simulink model "CubeSatTEST"  (R2024b)
settings: Solver=ode4  StartTime=simul.t0  StopTime=simul.tf  FixedStep=0.01  RelTol=1e-3
values from neighbouring files (symbols this model uses):
  alpha1 = 0.7    [mainSimTEST.m]
  alpha2 = 0.3    [mainSimTEST.m]
undefined symbols (not defined in the file or in its folder): act, DiscIntNeverNeededParam, env, flag, IC, K, orb, sat, sens
libraries: matrix_library x55, simulink_extras x5, simulink x2
(part 5 of 10)

== system CubeSatTEST/Real World/DKE (Dynamics Kinematics Environment)/Environment/Perturbations/Magnetic Field Torque ==
  r_n : Inport
  A(B/N) : Inport  Port=2
  Clock : Clock
  Constant : Constant  Value=env.mag.dgrf2020
  Constant1 : Constant  Value=env.Earth.R
  Constant2 : Constant  Value=3
  Constant3 : Constant  Value=env.Earth.magInclination
  Constant4 : Constant  Value=3
  Constant5 : Constant  Value=flag.mag
  Constant6 : Constant  Value=[0; 0; 0]
  Constant7 : Constant  Value=sat.jB
  Cos : Trigonometry  Operator=cos
  Cos1 : Trigonometry  Operator=cos
  Cross Product : matrix_library/Cross Product
  Divide : Product  Inputs=***/
  Divide1 : Product  Inputs=*/
  Divide2 : Product  Inputs=*/
  Dot Product : DotProduct  OutDataTypeStr=Inherit: Inherit via internal rule
  Gain : Gain  Gain=3
  Gain1 : Gain  Gain=env.Earth.omega
  Mux : Mux  Inputs=3
  Norm : Subsystem
  Norm1 : Subsystem
  Norm2 : Subsystem
  Power : Math  Operator=pow
  Power1 : Math  Operator=pow
  Product : Product
  Product1 : Product
  Product2 : Product
  Product9 : Product  Multiplication=Matrix(*)
  Sin : Trigonometry
  Sin1 : Trigonometry
  Sqrt : Sqrt
  Square : Math  Operator=square
  Subtract : Sum  Inputs=+-
  Sum of Elements : Sum  Inputs=+
  Switch : Switch  Criteria=u2 > Threshold  SaturateOnIntegerOverflow=off  InputSameDT=off
  T_mag : Outport
  wires:
  Constant/1 -> Square/1
  Square/1 -> Sum of Elements/1
  Sum of Elements/1 -> Sqrt/1
  Constant1/1 -> Power/1
  Constant2/1 -> Power/2
  Sqrt/1 -> Divide/2
  Power/1 -> Divide/3
  Constant4/1 -> Power1/2
  Power1/1 -> Divide/4
  Norm/1(Norm) -> Power1/1  "norm_r"
  r_n/1 -> Norm2/1(Vector), Divide2/1, [rr]
  [rr] -> Norm/1(Vector)
  [rr_hat] -> Dot Product/2
  Subtract/1 -> Divide/1
  [mm] -> Subtract/2
  Dot Product/1 -> Product/2
  Product/1 -> Gain/1
  Gain/1 -> Subtract/1
  [rr_hat] -> Product/1
  [mm] -> Dot Product/1
  Mux/1 -> Norm1/1(Vector), Divide1/1
  Cos/1 -> Mux/3
  Constant3/1 -> Sin/1, Cos/1
  Clock/1 -> Gain1/1
  Sin/1 -> Product2/2, Product1/2
  Product1/1 -> Mux/2
  Product2/1 -> Mux/1
  Cos1/1 -> Product2/1
  Gain1/1 -> Cos1/1, Sin1/1
  Sin1/1 -> Product1/1
  Divide/1 -> Product9/2
  Norm1/1(Norm) -> Divide1/2  "norm_r"
  Divide1/1 -> [mm]
  Norm2/1(Norm) -> Divide2/2  "norm_r"
  Divide2/1 -> [rr_hat]
  Constant5/1 -> Switch/2
  Constant6/1 -> Switch/3
  Cross Product/1 -> Switch/1
  A(B/N)/1 -> Product9/1
  Constant7/1 -> Cross Product/1
  Switch/1 -> T_mag/1
  Product9/1 -> Cross Product/2

== system CubeSatTEST/Real World/DKE (Dynamics Kinematics Environment)/Environment/Perturbations/Solar Radiation Pressure Torque ==
  S_b : Inport
  Constant : Constant  Value=flag.srp
  Constant1 : Constant  Value=[0; 0; 0]
  Constant3 : Constant  Value=ones(6,1)-sat.rho_s
  Constant4 : Constant  Value=sat.rho_s
  Constant5 : Constant  Value=sat.rho_d
  Gain1 : Gain  Gain=-env.dis.P
  Gain2 : Gain  Gain=2
  Gain3 : Gain  Gain=2/3
  Matrix Concatenate : Concatenate  NumInputs=3  Mode=Multidimensional array
  Matrix Concatenate2 : Concatenate  NumInputs=3  Mode=Multidimensional array
  MatrixMultiply : Product  Multiplication=Matrix(*)
  Normaliser : Subsystem
  Product{,1,3..4} (4 alike) : Product
  Product2 : Product  Multiplication=Matrix(*)
  Reshape : Reshape
  Saturation : Saturate  UpperLimit=1  LowerLimit=0
  Sum1 : Sum  Inputs=+|+
  Sum2 : Sum  Inputs=+|+
  Switch : Switch  Criteria=u2 > Threshold  SaturateOnIntegerOverflow=off  InputSameDT=off
  Transpose : Math  Operator=transpose
  Transpose2 : Math  Operator=transpose
  Transpose3 : Math  Operator=transpose
  cross product r x F : Subsystem
  surface : Constant  Value=sat.A
  unit vector matrix : Constant  Value=sat.n_b
  T_srp : Outport
  wires:
  Product3/1 -> Transpose3/1
  Saturation/1 -> Product4/2, Product1/1
  Gain3/1 -> Sum1/2
  surface/1 -> Gain1/1
  unit vector matrix/1 -> MatrixMultiply/2, Product/2
  Constant4/1 -> Gain2/1
  Constant3/1 -> Product2/1
  Sum2/1 -> Product3/2
  [S_b] -> Product2/2
  Constant5/1 -> Gain3/1
  Product4/1 -> Sum1/1
  MatrixMultiply/1 -> Saturation/1
  Gain2/1 -> Product4/1
  Product2/1 -> Transpose/1
  S_b/1 -> Normaliser/1(Vector)
  Normaliser/1(Out1) -> Transpose2/1
  Transpose2/1 -> MatrixMultiply/1, [S_b]
  Product/1 -> Sum2/2
  Transpose/1 -> Sum2/1
  Transpose3/1 -> cross product r x F/1(F_srp)
  Gain1/1 -> Product1/2
  Sum1/1 -> Matrix Concatenate/3, Matrix Concatenate/1, Matrix Concatenate/2
  Matrix Concatenate/1 -> Product/1
  Product1/1 -> Matrix Concatenate2/3, Matrix Concatenate2/2, Matrix Concatenate2/1
  Matrix Concatenate2/1 -> Product3/1
  cross product r x F/1(Out1) -> Switch/1
  Constant/1 -> Switch/2
  Switch/1 -> Reshape/1
  Constant1/1 -> Switch/3
  Reshape/1 -> T_srp/1

== system CubeSatTEST/Real World/DKE (Dynamics Kinematics Environment)/Environment/Sun Direction Circular Orbit/Normaliser (with Built In safety) ==
  Vector : Inport
  Constant : Constant  Value=[0; 0; 0]  VectorParams1D=off
  Norm1 : Subsystem
  Protected Division : Subsystem
  Switch : Switch  Criteria=u2 ~= 0  SaturateOnIntegerOverflow=off  InputSameDT=off
  Out1 : Outport
  wires:
  Norm1/1(Norm) -> Switch/2, Protected Division/2(Norm)  "norm_r"
  Switch/1 -> Out1/1
  Protected Division/1(Out1) -> Switch/1
  Vector/1 -> Protected Division/1(Vector), Norm1/1(Vector)
  Constant/1 -> Switch/3

== system CubeSatTEST/Real World/DKE (Dynamics Kinematics Environment)/Kinematics/EulerKinematicsdelay/312 Propagator ==
  IC : Inport
  w_b : Inport  Port=2
  Reset : Inport  Port=3
  Cos1 : Trigonometry  Operator=cos
  Cos2 : Trigonometry  Operator=cos
  Demux : Demux  Outputs=3
  Demux1 : Demux  Outputs=3
  Divide1 : Product  Inputs=*/
  Integrator1 : Integrator  ExternalReset=either  InitialConditionSource=external  WrapState=on  WrappedStateUpperValue=2*pi  WrappedStateLowerValue=0  ShowStatePort=on
  Integrator2 : Integrator  ExternalReset=either  InitialConditionSource=external  WrapState=on  ShowStatePort=on
  Integrator3 : Integrator  ExternalReset=either  InitialConditionSource=external  WrapState=on  WrappedStateUpperValue=2*pi  WrappedStateLowerValue=0  ShowStatePort=on
  Mux : Mux  Inputs=3
  Mux1 : Mux  Inputs=3
  Product{1..7} (7 alike) : Product
  Sin : Trigonometry
  Subtract : Sum  Inputs=+-
  Subtract1 : Sum
  Subtract2 : Sum  Inputs=+-
  Subtract3 : Sum  Inputs=+-
  Tan : Trigonometry  Operator=tan
  EA : Outport
  Out1 : Outport  Port=2
  wires:
  Product6/1 -> Subtract3/2
  Product5/1 -> Subtract3/1
  Product4/1 -> Subtract1/2
  Integrator3/1 -> [theta3]
  [wz] -> Product5/1
  Mux/1 -> EA/1
  Product7/1 -> Subtract2/2
  Cos1/1 -> [cosPsi]
  [theta3] -> Sin/1, Cos1/1
  [cosPsi] -> Product1/2
  Demux/2 -> [wy]
  Tan/1 -> [tanThe]
  Product2/1 -> Subtract/2
  [wz] -> Product3/1
  [tanThe] -> Product7/2
  Cos2/1 -> [cosThe]
  [cosPsi] -> Product5/2
  Divide1/1 -> Integrator1/1
  Subtract1/1 -> Integrator2/1
  Demux/3 -> [wz]
  [theta1] -> Mux/1
  Subtract/1 -> Divide1/1
  Demux/1 -> [wx]
  Subtract2/1 -> Integrator3/1
  [theta2] -> Tan/1, Cos2/1
  [wy] -> Subtract2/1
  Integrator1/1 -> [theta1]
  Integrator2/1 -> [theta2]
  [wx] -> Product4/1
  [sinPsi] -> Product2/2
  w_b/1 -> Demux/1
  Subtract3/1 -> Product7/1
  Product3/1 -> Subtract1/1
  [theta2] -> Mux/2
  [sinPsi] -> Product3/2
  [theta3] -> Mux/3
  [sinPsi] -> Product6/2
  [wx] -> Product6/1
  [wx] -> Product2/1
  [cosPsi] -> Product4/2
  [wz] -> Product1/1
  Product1/1 -> Subtract/1
  [cosThe] -> Divide1/2
  Sin/1 -> [sinPsi]
  Demux1/1 -> Integrator1/3
  Demux1/2 -> Integrator2/3
  Demux1/3 -> Integrator3/3
  IC/1 -> Demux1/1
  Reset/1 -> Integrator2/2, Integrator3/2, Integrator1/2
  Integrator3/State -> Mux1/3
  Integrator2/State -> Mux1/2
  Integrator1/State -> Mux1/1
  Mux1/1 -> Out1/1

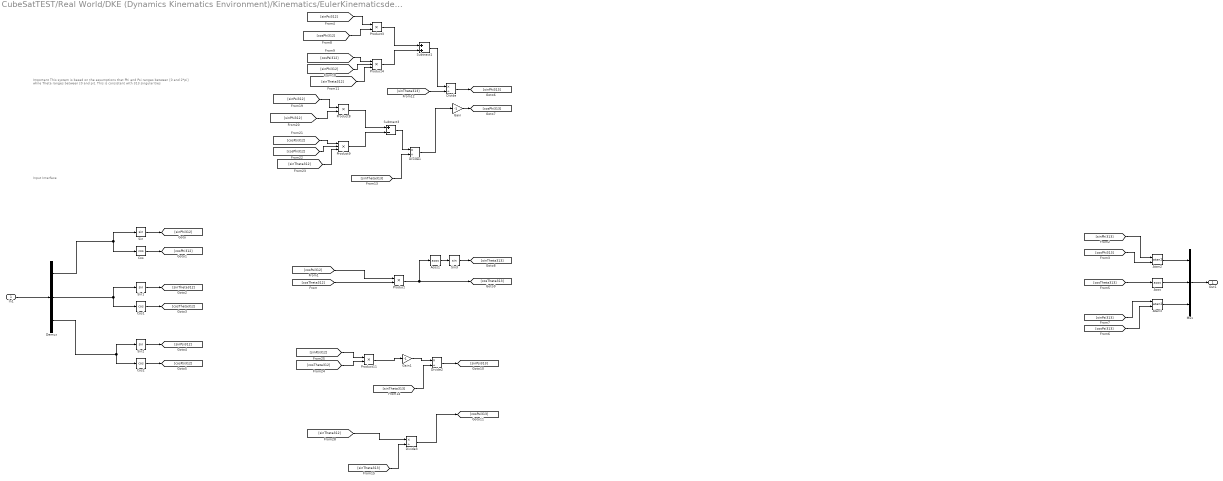
== system CubeSatTEST/Real World/DKE (Dynamics Kinematics Environment)/Kinematics/EulerKinematicsdelay/312To313 ==
  note: Important
      |
      | This system is based on the assumptions that Phi and Psi ranges between [0 and 2*pi] while Theta ranges between [0 and pi]. This is consistent with 313 singularities
  note: Input Interface
  In1 : Inport
  Acos : Trigonometry  Operator=acos
  Acos1 : Trigonometry  Operator=acos
  Atan2 : Trigonometry  Operator=atan2
  Atan3 : Trigonometry  Operator=atan2
  Cos : Trigonometry  Operator=cos
  Cos1 : Trigonometry  Operator=cos
  Cos2 : Trigonometry  Operator=cos
  Demux : Demux  Outputs=3
  Divide{,1..3} (4 alike) : Product  Inputs=*/
  Gain : Gain  Gain=-1
  Gain1 : Gain  Gain=-1
  Mux : Mux  Inputs=3
  Product{,3,8,11} (4 alike) : Product
  Product4 : Product  Inputs=3
  Product9 : Product  Inputs=3
  Sin{,1..3} (4 alike) : Trigonometry
  Subtract1 : Sum
  Subtract3 : Sum  Inputs=+-
  Out1 : Outport
  wires:
  In1/1 -> Demux/1
  Mux/1 -> Out1/1
  Sin/1 -> [sinPhi312]
  Cos/1 -> [cosPhi312]
  Demux/1 -> Sin/1, Cos/1
  Sin1/1 -> [sinTheta312]
  Demux/2 -> Sin1/1, Cos1/1
  Cos1/1 -> [cosTheta312]
  Sin2/1 -> [sinPsi312]
  Cos2/1 -> [cosPsi312]
  Demux/3 -> Sin2/1, Cos2/1
  Product/1 -> Acos1/1, [cosTheta313]
  [cosTheta312] -> Product/2
  [cosPsi312] -> Product/1
  Atan2/1 -> Mux/1
  Acos/1 -> Mux/2
  Atan3/1 -> Mux/3
  [sinPhi313] -> Atan2/1
  [cosPhi313] -> Atan2/2
  [cosTheta313] -> Acos/1
  [cosPsi313] -> Atan3/2
  [sinPsi313] -> Atan3/1
  Sin3/1 -> [sinTheta313]
  Acos1/1 -> Sin3/1
  [cosPsi312] -> Product4/1
  [sinTheta312] -> Product4/3
  Product3/1 -> Subtract1/1
  [cosPhi312] -> Product3/2
  Product4/1 -> Subtract1/2
  [sinPsi312] -> Product3/1
  [sinPhi312] -> Product4/2
  Divide/1 -> [sinPhi313]
  [sinTheta313] -> Divide/2
  Subtract1/1 -> Divide/1
  Gain/1 -> [cosPhi313]
  Divide1/1 -> Gain/1
  [sinTheta313] -> Divide1/2
  [cosPsi312] -> Product9/1
  Product9/1 -> Subtract3/2
  Subtract3/1 -> Divide1/1
  [sinPsi312] -> Product8/1
  [cosPhi312] -> Product9/2
  [sinPhi312] -> Product8/2
  [sinTheta312] -> Product9/3
  Product8/1 -> Subtract3/1
  [sinTheta313] -> Divide2/2
  Divide2/1 -> [sinPsi313]
  [sinTheta313] -> Divide3/2
  Divide3/1 -> [cosPsi313]
  Product11/1 -> Gain1/1
  [sinPsi312] -> Product11/1
  [cosTheta312] -> Product11/2
  Gain1/1 -> Divide2/1
  [sinTheta312] -> Divide3/1

== system CubeSatTEST/Real World/DKE (Dynamics Kinematics Environment)/Kinematics/EulerKinematicsdelay/313 Propagator ==
  note: Phi
  note: Theta
  Reset : Inport
  w_b : Inport  Port=2
  IC : Inport  Port=3
  Cos1 : Trigonometry  Operator=cos
  Cos2 : Trigonometry
  Demux : Demux  Outputs=3
  Demux1 : Demux  Outputs=3
  Divide : Product  Inputs=/
  Divide1 : Product  Inputs=*/
  Integrator1 : Integrator  ExternalReset=either  InitialConditionSource=external  WrapState=on  WrappedStateUpperValue=2*pi  WrappedStateLowerValue=0  ShowStatePort=on
  Integrator2 : Integrator  ExternalReset=either  InitialConditionSource=external  InitialCondition=pi/4  WrapState=on  ShowStatePort=on
  Integrator3 : Integrator  ExternalReset=either  InitialConditionSource=external  WrapState=on  WrappedStateUpperValue=2*pi  WrappedStateLowerValue=0  ShowStatePort=on
  Mux : Mux  Inputs=3
  Mux1 : Mux  Inputs=3
  Product{1..7} (7 alike) : Product
  Sin : Trigonometry
  Subtract : Sum
  Subtract1 : Sum  Inputs=-+
  Subtract2 : Sum  Inputs=+-
  Subtract3 : Sum
  Tan : Trigonometry  Operator=tan
  EA : Outport
  Out1 : Outport  Port=2
  wires:
  [sinThe] -> Divide1/2
  Sin/1 -> [sinPsi]
  [wx] -> Product2/1
  [theta3] -> Mux/3
  [theta2] -> Mux/2
  Product3/1 -> Subtract1/1
  w_b/1 -> Demux/1
  [sinPsi] -> Product3/2
  [sinPsi] -> Product6/2
  Subtract3/1 -> Product7/1
  Product1/1 -> Subtract/1
  [wx] -> Product6/1
  [wy] -> Product1/1
  [wz] -> Subtract2/1
  Subtract2/1 -> Integrator3/1
  [theta2] -> Tan/1, Cos2/1
  [cosPsi] -> Product4/2
  Demux/1 -> [wx]
  [sinPsi] -> Product2/2
  Integrator2/1 -> [theta2]
  [wx] -> Product4/1
  Tan/1 -> Divide/1
  [cosPsi] -> Product1/2
  Divide1/1 -> Integrator1/1
  Integrator1/1 -> [theta1]
  [ctanThe] -> Product7/2
  [cosPsi] -> Product5/2
  [wy] -> Product3/1
  Product2/1 -> Subtract/2
  Demux/2 -> [wy]
  Product5/1 -> Subtract3/1
  [wy] -> Product5/1
  Integrator3/1 -> [theta3]
  Product6/1 -> Subtract3/2
  Mux/1 -> EA/1
  Product4/1 -> Subtract1/2
  [theta3] -> Sin/1, Cos1/1
  Product7/1 -> Subtract2/2
  Cos2/1 -> [sinThe]
  Subtract1/1 -> Integrator2/1
  [theta1] -> Mux/1
  Subtract/1 -> Divide1/1
  Demux/3 -> [wz]
  Cos1/1 -> [cosPsi]
  Divide/1 -> [ctanThe]
  Demux1/3 -> Integrator3/3
  Demux1/2 -> Integrator2/3
  Demux1/1 -> Integrator1/3
  IC/1 -> Demux1/1
  Reset/1 -> Integrator1/2, Integrator2/2, Integrator3/2
  Integrator3/State -> Mux1/3
  Integrator2/State -> Mux1/2
  Mux1/1 -> Out1/1
  Integrator1/State -> Mux1/1

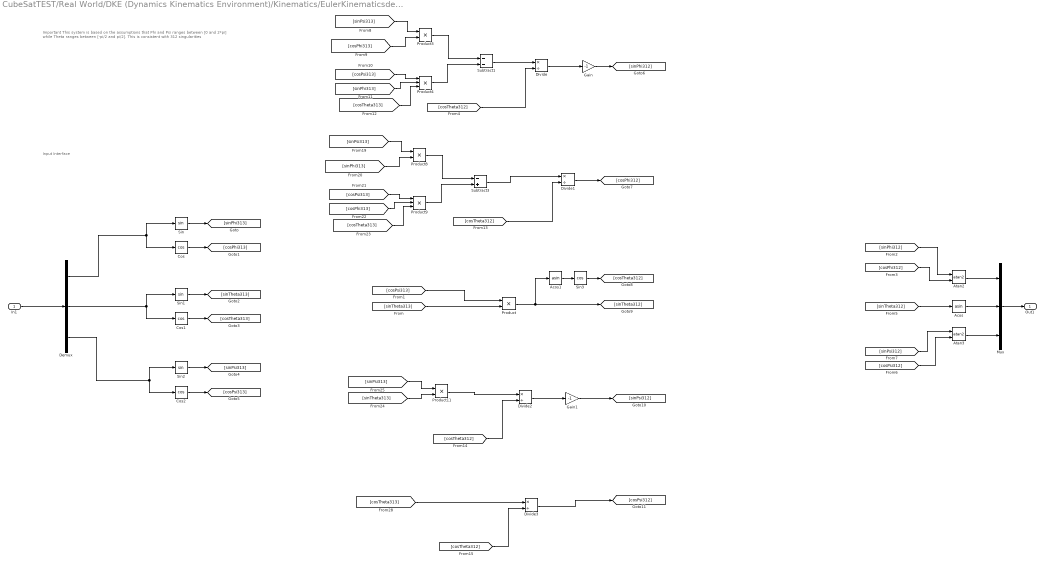
== system CubeSatTEST/Real World/DKE (Dynamics Kinematics Environment)/Kinematics/EulerKinematicsdelay/313To312 ==
  note: Input Interface
  note: Important
      |
      | This system is based on the assumptions that Phi and Psi ranges between [0 and 2*pi] while Theta ranges between [-pi/2 and pi/2]. This is consistent with 312 singularities
  In1 : Inport
  Acos : Trigonometry  Operator=asin
  Acos1 : Trigonometry  Operator=asin
  Atan2 : Trigonometry  Operator=atan2
  Atan3 : Trigonometry  Operator=atan2
  Cos : Trigonometry  Operator=cos
  Cos1 : Trigonometry  Operator=cos
  Cos2 : Trigonometry  Operator=cos
  Demux : Demux  Outputs=3
  Divide{,1..3} (4 alike) : Product  Inputs=*/
  Gain : Gain  Gain=-1
  Gain1 : Gain  Gain=-1
  Mux : Mux  Inputs=3
  Product{,3,8,11} (4 alike) : Product
  Product4 : Product  Inputs=3
  Product9 : Product  Inputs=3
  Sin : Trigonometry
  Sin1 : Trigonometry
  Sin2 : Trigonometry
  Sin3 : Trigonometry  Operator=cos
  Subtract1 : Sum  Inputs=--
  Subtract3 : Sum  Inputs=-+
  Out1 : Outport
  wires:
  Cos/1 -> [cosPhi313]
  Sin/1 -> [sinPhi313]
  Cos1/1 -> [cosTheta313]
  Demux/3 -> Sin2/1, Cos2/1
  Demux/1 -> Sin/1, Cos/1
  Sin2/1 -> [sinPsi313]
  Sin1/1 -> [sinTheta313]
  In1/1 -> Demux/1
  Demux/2 -> Sin1/1, Cos1/1
  Cos2/1 -> [cosPsi313]
  Mux/1 -> Out1/1
  [sinTheta312] -> Acos/1
  Atan3/1 -> Mux/3
  Atan2/1 -> Mux/1
  [sinPhi312] -> Atan2/1
  [cosPhi312] -> Atan2/2
  [sinPsi312] -> Atan3/1
  [cosPsi312] -> Atan3/2
  Acos/1 -> Mux/2
  [sinTheta313] -> Product/2
  Product/1 -> Acos1/1, [sinTheta312]
  Sin3/1 -> [cosTheta312]
  [cosPsi313] -> Product/1
  Acos1/1 -> Sin3/1
  Gain/1 -> [sinPhi312]
  Divide/1 -> Gain/1
  [cosTheta312] -> Divide/2
  Product3/1 -> Subtract1/1
  [cosPhi313] -> Product3/2
  Product4/1 -> Subtract1/2
  [cosPsi313] -> Product4/1
  [sinPhi313] -> Product4/2
  Subtract1/1 -> Divide/1
  [sinPsi313] -> Product3/1
  [cosTheta313] -> Product4/3
  [cosTheta312] -> Divide1/2
  Divide1/1 -> [cosPhi312]
  [cosPsi313] -> Product9/1
  Product9/1 -> Subtract3/2
  [sinPsi313] -> Product8/1
  [sinPhi313] -> Product8/2
  Product8/1 -> Subtract3/1
  [cosTheta313] -> Product9/3
  Subtract3/1 -> Divide1/1
  [cosPhi313] -> Product9/2
  Divide2/1 -> Gain1/1
  [cosTheta312] -> Divide2/2
  Gain1/1 -> [sinPsi312]
  [sinTheta313] -> Product11/2
  Product11/1 -> Divide2/1
  [sinPsi313] -> Product11/1
  [cosTheta312] -> Divide3/2
  [cosTheta313] -> Divide3/1
  Divide3/1 -> [cosPsi312]

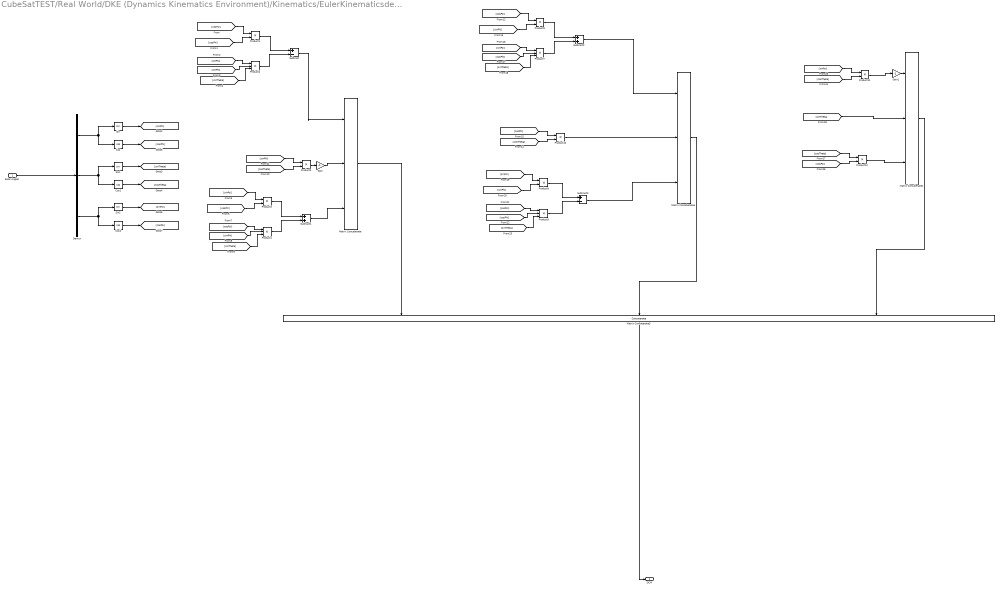
== system CubeSatTEST/Real World/DKE (Dynamics Kinematics Environment)/Kinematics/EulerKinematicsdelay/A312 ==
  Euler Angles : Inport
  Cos : Trigonometry  Operator=cos
  Cos1 : Trigonometry  Operator=cos
  Cos2 : Trigonometry  Operator=cos
  Demux : Demux  Outputs=3
  Gain : Gain  Gain=-1
  Gain1 : Gain  Gain=-1
  Matrix Concatenate : Concatenate  NumInputs=3  Mode=Multidimensional array
  Matrix Concatenate1 : Concatenate  NumInputs=3  Mode=Multidimensional array
  Matrix Concatenate3 : Concatenate  NumInputs=3  Mode=Multidimensional array  ConcatenateDimension=2
  Matrix Concatenate4 : Concatenate  NumInputs=3  Mode=Multidimensional array
  Product{1,3,5..6,8,10..12} (8 alike) : Product
  Product{2,4,7,9} (4 alike) : Product  Inputs=3
  Sin : Trigonometry
  Sin1 : Trigonometry
  Sin2 : Trigonometry
  Subtract : Sum  Inputs=+-
  Subtract1 : Sum
  Subtract2 : Sum
  Subtract3 : Sum  Inputs=+-
  DCM : Outport
  wires:
  Euler Angles/1 -> Demux/1
  [sinTheta] -> Product2/3
  Product7/1 -> Subtract2/2
  [cosTheta] -> Product11/2
  [sinPhi] -> Product8/2
  Sin/1 -> [sinPhi]
  [sinPhi] -> Product2/2
  [cosTheta] -> Product10/2
  [cosPsi] -> Product6/1
  Demux/3 -> Sin2/1, Cos2/1
  Product9/1 -> Subtract3/2
  [sinTheta] -> Matrix Concatenate1/2
  Matrix Concatenate1/1 -> Matrix Concatenate3/3
  [sinPsi] -> Product11/1
  Product2/1 -> Subtract/2
  Subtract2/1 -> Matrix Concatenate4/1
  Matrix Concatenate4/1 -> Matrix Concatenate3/2
  [cosTheta] -> Product12/1
  Cos2/1 -> [cosPsi]
  [sinPsi] -> Product2/1
  [sinPsi] -> Product8/1
  Sin2/1 -> [sinPsi]
  [sinTheta] -> Product7/3
  Subtract/1 -> Matrix Concatenate/1
  [cosPhi] -> Product10/1
  Demux/2 -> Sin1/1, Cos1/1
  [sinTheta] -> Product9/3
  Product8/1 -> Subtract3/1
  [cosPhi] -> Product9/2
  [cosPsi] -> Product9/1
  Product11/1 -> Gain1/1
  Product1/1 -> Subtract/1
  [cosPhi] -> Product1/2
  [cosPsi] -> Product12/2
  [cosPhi] -> Product7/2
  [sinPhi] -> Product6/2
  Product6/1 -> Subtract2/1
  Demux/1 -> Sin/1, Cos/1
  [cosPsi] -> Product1/1
  [sinPsi] -> Product7/1
  Cos1/1 -> [cosTheta]
  Sin1/1 -> [sinTheta]
  Product12/1 -> Matrix Concatenate1/3
  Matrix Concatenate/1 -> Matrix Concatenate3/1
  Cos/1 -> [cosPhi]
  Matrix Concatenate3/1 -> DCM/1
  Gain1/1 -> Matrix Concatenate1/1
  Product10/1 -> Matrix Concatenate4/2
  Subtract3/1 -> Matrix Concatenate4/3
  [cosPsi] -> Product4/1
  Product4/1 -> Subtract1/2
  [cosPhi] -> Product3/2
  Product3/1 -> Subtract1/1
  [sinPsi] -> Product3/1
  [sinPhi] -> Product4/2
  [sinTheta] -> Product4/3
  [sinPhi] -> Product5/1
  [cosTheta] -> Product5/2
  Product5/1 -> Gain/1
  Subtract1/1 -> Matrix Concatenate/3
  Gain/1 -> Matrix Concatenate/2

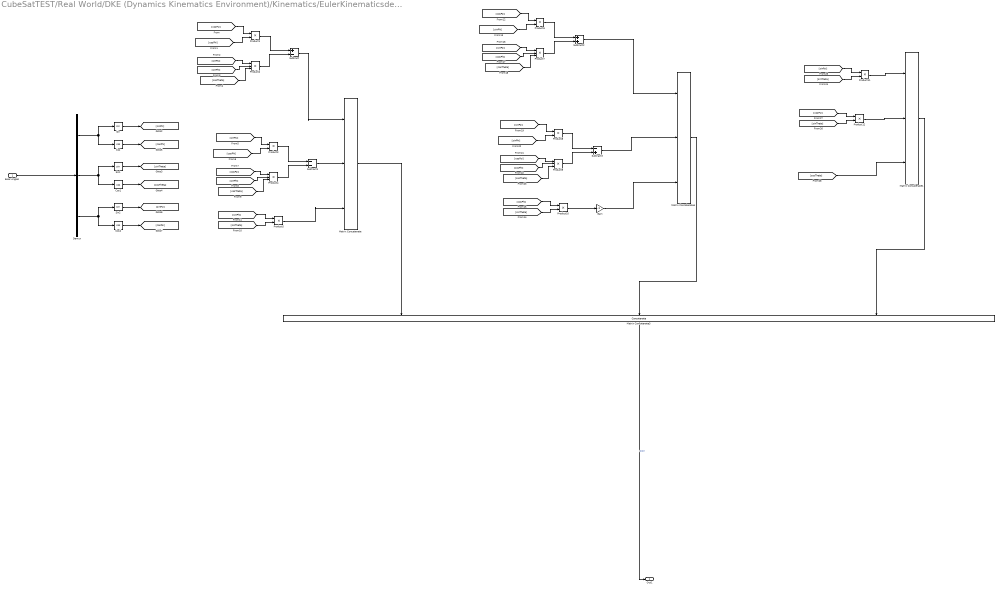
== system CubeSatTEST/Real World/DKE (Dynamics Kinematics Environment)/Kinematics/EulerKinematicsdelay/A313 ==
  Euler Angles : Inport
  Cos : Trigonometry  Operator=cos
  Cos1 : Trigonometry  Operator=cos
  Cos2 : Trigonometry  Operator=cos
  Demux : Demux  Outputs=3
  Gain : Gain  Gain=-1
  Matrix Concatenate : Concatenate  NumInputs=3  Mode=Multidimensional array
  Matrix Concatenate1 : Concatenate  NumInputs=3  Mode=Multidimensional array
  Matrix Concatenate3 : Concatenate  NumInputs=3  Mode=Multidimensional array  ConcatenateDimension=2
  Matrix Concatenate4 : Concatenate  NumInputs=3  Mode=Multidimensional array
  Product{1,3,5..6,8,10..12} (8 alike) : Product
  Product{2,4,7,9} (4 alike) : Product  Inputs=3
  Sin : Trigonometry
  Sin1 : Trigonometry
  Sin2 : Trigonometry
  Subtract : Sum  Inputs=+-
  Subtract1 : Sum  Inputs=--
  Subtract2 : Sum
  Subtract3 : Sum  Inputs=-+
  Out1 : Outport
  wires:
  Euler Angles/1 -> Demux/1
  [cosTheta] -> Product2/3
  Product7/1 -> Subtract2/2
  [sinTheta] -> Product11/2
  [sinPhi] -> Product8/2
  Sin/1 -> [sinPhi]
  [cosTheta] -> Product4/3
  [sinPhi] -> Product2/2
  [sinTheta] -> Product10/2
  Product5/1 -> Matrix Concatenate/3
  [cosPsi] -> Product6/1
  Demux/3 -> Sin2/1, Cos2/1
  Product9/1 -> Subtract3/2
  [cosTheta] -> Matrix Concatenate1/3
  Matrix Concatenate1/1 -> Matrix Concatenate3/3
  [sinPsi] -> Product11/1
  Product2/1 -> Subtract/2
  [sinPhi] -> Product4/2
  Subtract2/1 -> Matrix Concatenate4/1
  Matrix Concatenate4/1 -> Matrix Concatenate3/2
  [cosPsi] -> Product12/1
  Cos2/1 -> [cosPsi]
  Product10/1 -> Gain/1
  [sinPsi] -> Product2/1
  [sinPsi] -> Product8/1
  Sin2/1 -> [sinPsi]
  [cosTheta] -> Product7/3
  Subtract/1 -> Matrix Concatenate/1
  [cosPhi] -> Product10/1
  Subtract1/1 -> Matrix Concatenate/2
  Subtract3/1 -> Matrix Concatenate4/2
  Demux/2 -> Sin1/1, Cos1/1
  [cosTheta] -> Product9/3
  Product8/1 -> Subtract3/1
  [cosPhi] -> Product9/2
  [cosPsi] -> Product9/1
  Gain/1 -> Matrix Concatenate4/3
  [cosPsi] -> Product4/1
  Product11/1 -> Matrix Concatenate1/1
  Product1/1 -> Subtract/1
  [cosPhi] -> Product1/2
  [sinTheta] -> Product12/2
  [cosPhi] -> Product7/2
  [sinPhi] -> Product6/2
  Product6/1 -> Subtract2/1
  Demux/1 -> Sin/1, Cos/1
  [cosPsi] -> Product1/1
  [sinPsi] -> Product7/1
  Cos1/1 -> [cosTheta]
  Sin1/1 -> [sinTheta]
  [sinTheta] -> Product5/2
  [sinPsi] -> Product3/1
  Product12/1 -> Matrix Concatenate1/2
  [sinPhi] -> Product5/1
  Product3/1 -> Subtract1/1
  Product4/1 -> Subtract1/2
  [cosPhi] -> Product3/2
  Matrix Concatenate/1 -> Matrix Concatenate3/1
  Cos/1 -> [cosPhi]
  Matrix Concatenate3/1 -> Out1/1  "DCM"

== system CubeSatTEST/Real World/Hardware Models/Actuators/CMG + Control Logic/A assembler ==
  delta : Inport
  beta : Inport  Port=2
  Cos : Trigonometry  Operator=cos
  Cos1 : Trigonometry  Operator=cos
  Gain{,1..3} (4 alike) : Gain  Gain=-1
  Matrix Concatenate : Concatenate  NumInputs=4  Mode=Multidimensional array  ConcatenateDimension=2
  Matrix Concatenate{1..4} (4 alike) : Concatenate  NumInputs=3  Mode=Multidimensional array
  Product{,1..7} (8 alike) : Product
  Selector : Selector  InputPortWidth=4  IndexOptions=Index vector (dialog)  Indices=1  OutputSizes=1
  Selector1 : Selector  InputPortWidth=4  IndexOptions=Index vector (dialog)  Indices=1  OutputSizes=1
  Selector10 : Selector  InputPortWidth=4  IndexOptions=Index vector (dialog)  Indices=4  OutputSizes=1
  Selector11 : Selector  InputPortWidth=4  IndexOptions=Index vector (dialog)  Indices=4  OutputSizes=1
  Selector2 : Selector  InputPortWidth=4  IndexOptions=Index vector (dialog)  Indices=1  OutputSizes=1
  Selector3 : Selector  InputPortWidth=4  IndexOptions=Index vector (dialog)  Indices=2  OutputSizes=1
  Selector4 : Selector  InputPortWidth=4  IndexOptions=Index vector (dialog)  Indices=2  OutputSizes=1
  Selector5 : Selector  InputPortWidth=4  IndexOptions=Index vector (dialog)  Indices=2  OutputSizes=1
  Selector6 : Selector  InputPortWidth=4  IndexOptions=Index vector (dialog)  Indices=3  OutputSizes=1
  Selector7 : Selector  InputPortWidth=4  IndexOptions=Index vector (dialog)  Indices=3  OutputSizes=1
  Selector8 : Selector  InputPortWidth=4  IndexOptions=Index vector (dialog)  Indices=3  OutputSizes=1
  Selector9 : Selector  InputPortWidth=4  IndexOptions=Index vector (dialog)  Indices=4  OutputSizes=1
  Sin : Trigonometry
  Sin1 : Trigonometry
  A : Outport
  wires:
  delta/1 -> Cos/1, Sin/1
  Cos/1 -> [cosd]
  Sin/1 -> [sind]
  Cos1/1 -> [cosb]
  Sin1/1 -> [sinb]
  beta/1 -> Sin1/1, Cos1/1
  Gain/1 -> Matrix Concatenate1/1
  Gain1/1 -> Matrix Concatenate2/1
  Gain2/1 -> Matrix Concatenate2/2
  Gain3/1 -> Matrix Concatenate3/2
  Matrix Concatenate1/1 -> Matrix Concatenate/1
  Matrix Concatenate2/1 -> Matrix Concatenate/2
  Matrix Concatenate3/1 -> Matrix Concatenate/3
  Matrix Concatenate4/1 -> Matrix Concatenate/4
  Matrix Concatenate/1 -> A/1
  Product/1 -> Gain/1
  Product1/1 -> Matrix Concatenate1/3
  Product2/1 -> Gain2/1
  Product3/1 -> Matrix Concatenate2/3
  Product4/1 -> Matrix Concatenate3/1
  Product5/1 -> Matrix Concatenate3/3
  Product6/1 -> Matrix Concatenate4/2
  Product7/1 -> Matrix Concatenate4/3
  [cosb] -> Product/1
  [cosb] -> Product2/1
  [cosb] -> Product4/1
  [cosb] -> Product6/1
  [sinb] -> Product1/1
  [sinb] -> Product3/1
  [sinb] -> Product5/1
  [sinb] -> Product7/1
  Selector/1 -> Matrix Concatenate1/2
  Selector1/1 -> Product/2
  Selector2/1 -> Product1/2
  Selector3/1 -> Gain1/1
  Selector4/1 -> Product2/2
  Selector5/1 -> Product3/2
  Selector6/1 -> Product5/2
  Selector7/1 -> Gain3/1
  Selector8/1 -> Product4/2
  Selector9/1 -> Matrix Concatenate4/1
  Selector10/1 -> Product6/2
  Selector11/1 -> Product7/2
  [sind] -> Selector1/1
  [sind] -> Selector2/1
  [cosd] -> Selector/1
  [cosd] -> Selector3/1
  [cosd] -> Selector7/1
  [cosd] -> Selector9/1
  [sind] -> Selector5/1
  [sind] -> Selector4/1
  [sind] -> Selector6/1
  [sind] -> Selector8/1
  [sind] -> Selector10/1
  [sind] -> Selector11/1

== system CubeSatTEST/Real World/Hardware Models/Actuators/CMG + Control Logic/B assembler ==
  beta : Inport
  delta : Inport  Port=2
  Cos : Trigonometry  Operator=cos
  Cos1 : Trigonometry  Operator=cos
  Gain{,1..3} (4 alike) : Gain  Gain=-1
  Matrix Concatenate : Concatenate  NumInputs=4  Mode=Multidimensional array  ConcatenateDimension=2
  Matrix Concatenate{1..4} (4 alike) : Concatenate  NumInputs=3  Mode=Multidimensional array
  Product{,1..7} (8 alike) : Product
  Selector : Selector  InputPortWidth=4  IndexOptions=Index vector (dialog)  Indices=1  OutputSizes=1
  Selector1 : Selector  InputPortWidth=4  IndexOptions=Index vector (dialog)  Indices=1  OutputSizes=1
  Selector10 : Selector  InputPortWidth=4  IndexOptions=Index vector (dialog)  Indices=4  OutputSizes=1
  Selector11 : Selector  InputPortWidth=4  IndexOptions=Index vector (dialog)  Indices=4  OutputSizes=1
  Selector2 : Selector  InputPortWidth=4  IndexOptions=Index vector (dialog)  Indices=1  OutputSizes=1
  Selector3 : Selector  InputPortWidth=4  IndexOptions=Index vector (dialog)  Indices=2  OutputSizes=1
  Selector4 : Selector  InputPortWidth=4  IndexOptions=Index vector (dialog)  Indices=2  OutputSizes=1
  Selector5 : Selector  InputPortWidth=4  IndexOptions=Index vector (dialog)  Indices=2  OutputSizes=1
  Selector6 : Selector  InputPortWidth=4  IndexOptions=Index vector (dialog)  Indices=3  OutputSizes=1
  Selector7 : Selector  InputPortWidth=4  IndexOptions=Index vector (dialog)  Indices=3  OutputSizes=1
  Selector8 : Selector  InputPortWidth=4  IndexOptions=Index vector (dialog)  Indices=3  OutputSizes=1
  Selector9 : Selector  InputPortWidth=4  IndexOptions=Index vector (dialog)  Indices=4  OutputSizes=1
  Sin : Trigonometry
  Sin1 : Trigonometry
  B : Outport
  wires:
  Cos/1 -> [cosd]
  Sin/1 -> [sind]
  delta/1 -> Cos/1, Sin/1
  beta/1 -> Sin1/1, Cos1/1
  Sin1/1 -> [sinb]
  Cos1/1 -> [cosb]
  Gain/1 -> Matrix Concatenate1/1
  Gain1/1 -> Matrix Concatenate1/2
  Gain2/1 -> Matrix Concatenate2/2
  Gain3/1 -> Matrix Concatenate4/1
  Matrix Concatenate1/1 -> Matrix Concatenate/1
  Matrix Concatenate2/1 -> Matrix Concatenate/2
  Matrix Concatenate3/1 -> Matrix Concatenate/3
  Matrix Concatenate4/1 -> Matrix Concatenate/4
  Matrix Concatenate/1 -> B/1
  Product/1 -> Gain/1
  Product1/1 -> Matrix Concatenate1/3
  Product2/1 -> Gain2/1
  Product3/1 -> Matrix Concatenate2/3
  Product4/1 -> Matrix Concatenate3/1
  Product5/1 -> Matrix Concatenate3/3
  Product6/1 -> Matrix Concatenate4/2
  Product7/1 -> Matrix Concatenate4/3
  Selector/1 -> Gain1/1
  Selector1/1 -> Product1/2
  Selector2/1 -> Product/2
  Selector3/1 -> Matrix Concatenate2/1
  Selector4/1 -> Product2/1
  Selector5/1 -> Product3/2
  Selector6/1 -> Product5/2
  Selector7/1 -> Matrix Concatenate3/2
  Selector8/1 -> Product4/1
  Selector9/1 -> Gain3/1
  Selector10/1 -> Product6/2
  Selector11/1 -> Product7/2
  [sind] -> Selector/1
  [sind] -> Selector3/1
  [sind] -> Selector7/1
  [sind] -> Selector9/1
  [cosd] -> Selector2/1
  [cosd] -> Selector1/1
  [cosd] -> Selector5/1
  [cosd] -> Selector4/1
  [cosd] -> Selector8/1
  [cosd] -> Selector6/1
  [cosd] -> Selector11/1
  [cosd] -> Selector10/1
  [cosb] -> Product/1
  [cosb] -> Product2/2
  [cosb] -> Product4/2
  [cosb] -> Product6/1
  [sinb] -> Product1/1
  [sinb] -> Product3/1
  [sinb] -> Product5/1
  [sinb] -> Product7/1

== system CubeSatTEST/Real World/Hardware Models/Actuators/CMG + Control Logic/CMG ==
  delta_dot : Inport
  w : Inport  Port=2
  Dynamics : Subsystem
  Quantizer : Quantizer  Commented=through  QuantizationInterval=act.cmg.quanta
  Saturation : Saturate  UpperLimit=act.cmg.sat  LowerLimit=-act.cmg.sat  LinearizeAsGain=off
  State : Subsystem
  delta : Outport
  Mc : Outport  Port=2
  wires:
  Dynamics/1(Mc) -> Saturation/1
  State/2(A) -> Dynamics/1(A)
  State/3(B) -> Dynamics/2(B)
  w/1 -> Dynamics/4(w)
  State/1(delta) -> Quantizer/1
  Quantizer/1 -> delta/1
  delta_dot/1 -> Dynamics/3(delta_dot), State/1(delta_dot)
  Saturation/1 -> Mc/1

== system CubeSatTEST/Real World/Hardware Models/Sensors/MAGNETOMETER/Noise x ==
  Bx_real : Inport
  Gain : Gain  Gain=1/sens.mag.SNR
  Product : Product
  Sqrt : Sqrt
  Square : Math  Operator=square
  white noise : RandomNumber  SampleTime=sens.mag.Ts
  Out1 : Outport
  wires:
  Product/1 -> Out1/1
  Sqrt/1 -> Product/1
  Gain/1 -> Sqrt/1
  white noise/1 -> Product/2
  Square/1 -> Gain/1
  Bx_real/1 -> Square/1

== system CubeSatTEST/Real World/Hardware Models/Sensors/MAGNETOMETER/Noise y ==
  By_real : Inport
  Gain : Gain  Gain=1/sens.mag.SNR
  Product : Product
  Sqrt : Sqrt
  Square : Math  Operator=square
  white noise : RandomNumber  SampleTime=sens.mag.Ts
  Out1 : Outport
  wires:
  Product/1 -> Out1/1
  Sqrt/1 -> Product/1
  Gain/1 -> Sqrt/1
  white noise/1 -> Product/2
  Square/1 -> Gain/1
  By_real/1 -> Square/1

== system CubeSatTEST/Real World/Hardware Models/Sensors/MAGNETOMETER/Noise z ==
  Bz_real : Inport
  Gain : Gain  Gain=1/sens.mag.SNR
  Product : Product
  Sqrt : Sqrt
  Square : Math  Operator=square
  white noise : RandomNumber  SampleTime=sens.mag.Ts
  Out1 : Outport
  wires:
  Product/1 -> Out1/1
  Sqrt/1 -> Product/1
  Gain/1 -> Sqrt/1
  white noise/1 -> Product/2
  Square/1 -> Gain/1
  Bz_real/1 -> Square/1

== system CubeSatTEST/Real World/Hardware Models/Sensors/SS Selector/Norm1 ==
  Vector : Inport
  Add : Sum  Inputs=+++
  Demux : Demux  Outputs=3
  Sqrt : Sqrt
  Square : Math  Operator=square
  Square1 : Math  Operator=square
  Square2 : Math  Operator=square
  Norm : Outport
  wires:
  Square/1 -> Add/1
  Add/1 -> Sqrt/1
  Demux/3 -> Square1/1
  Square2/1 -> Add/2
  Square1/1 -> Add/3
  Demux/1 -> Square/1
  Demux/2 -> Square2/1
  Vector/1 -> Demux/1
  Sqrt/1 -> Norm/1

== system CubeSatTEST/Real World/Hardware Models/Sensors/SS Selector/Norm2 ==
  Vector : Inport
  Add : Sum  Inputs=+++
  Demux : Demux  Outputs=3
  Sqrt : Sqrt
  Square : Math  Operator=square
  Square1 : Math  Operator=square
  Square2 : Math  Operator=square
  Norm : Outport
  wires:
  Square/1 -> Add/1
  Add/1 -> Sqrt/1
  Demux/3 -> Square1/1
  Square2/1 -> Add/2
  Square1/1 -> Add/3
  Demux/1 -> Square/1
  Demux/2 -> Square2/1
  Vector/1 -> Demux/1
  Sqrt/1 -> Norm/1

== system CubeSatTEST/Real World/Hardware Models/Sensors/SS Selector/Norm3 ==
  Vector : Inport
  Add : Sum  Inputs=+++
  Demux : Demux  Outputs=3
  Sqrt : Sqrt
  Square : Math  Operator=square
  Square1 : Math  Operator=square
  Square2 : Math  Operator=square
  Norm : Outport
  wires:
  Square/1 -> Add/1
  Add/1 -> Sqrt/1
  Demux/3 -> Square1/1
  Square2/1 -> Add/2
  Square1/1 -> Add/3
  Demux/1 -> Square/1
  Demux/2 -> Square2/1
  Vector/1 -> Demux/1
  Sqrt/1 -> Norm/1

== system CubeSatTEST/Real World/Hardware Models/Sensors/SS Selector/Norm4 ==
  Vector : Inport
  Add : Sum  Inputs=+++
  Demux : Demux  Outputs=3
  Sqrt : Sqrt
  Square : Math  Operator=square
  Square1 : Math  Operator=square
  Square2 : Math  Operator=square
  Norm : Outport
  wires:
  Square/1 -> Add/1
  Add/1 -> Sqrt/1
  Demux/3 -> Square1/1
  Square2/1 -> Add/2
  Square1/1 -> Add/3
  Demux/1 -> Square/1
  Demux/2 -> Square2/1
  Vector/1 -> Demux/1
  Sqrt/1 -> Norm/1

== system CubeSatTEST/Real World/Hardware Models/Sensors/Sun Sensor (Fine)/Mesurable (1) ==
  Action Port : ActionPort  ActionPortLabel=if((u1 == 0) & (u2 >= u3))
  Constant : Constant
  One : Outport
  wires:
  Constant/1 -> One/1

== system CubeSatTEST/Real World/Hardware Models/Sensors/Sun Sensor (Fine)/Not Mesurable (0) ==
  Action Port : ActionPort  ActionPortLabel=else
  Constant : Constant  Value=0
  Zero : Outport
  wires:
  Constant/1 -> Zero/1

== system CubeSatTEST/Real World/Hardware Models/Sensors/Sun Sensor (S1)/Mesurable (1) ==
  Action Port : ActionPort  ActionPortLabel=if((u1 == 0) & (u2 >= u3))
  Constant : Constant
  One : Outport
  wires:
  Constant/1 -> One/1

== system CubeSatTEST/Real World/Hardware Models/Sensors/Sun Sensor (S1)/Not Mesurable (0) ==
  Action Port : ActionPort  ActionPortLabel=else
  Constant : Constant  Value=0
  Zero : Outport
  wires:
  Constant/1 -> Zero/1

== system CubeSatTEST/Real World/Hardware Models/Sensors/Sun Sensor (S2)/Mesurable (1) ==
  Action Port : ActionPort  ActionPortLabel=if((u1 == 0) & (u2 >= u3))
  Constant : Constant
  One : Outport
  wires:
  Constant/1 -> One/1

== system CubeSatTEST/Real World/Hardware Models/Sensors/Sun Sensor (S2)/Not Mesurable (0) ==
  Action Port : ActionPort  ActionPortLabel=else
  Constant : Constant  Value=0
  Zero : Outport
  wires:
  Constant/1 -> Zero/1

== system CubeSatTEST/Real World/Hardware Models/Sensors/Sun Sensor (S3)/Mesurable (1) ==
  Action Port : ActionPort  ActionPortLabel=if((u1 == 0) & (u2 >= u3))
  Constant : Constant
  One : Outport
  wires:
  Constant/1 -> One/1

== system CubeSatTEST/Real World/Hardware Models/Sensors/Sun Sensor (S3)/Not Mesurable (0) ==
  Action Port : ActionPort  ActionPortLabel=else
  Constant : Constant  Value=0
  Zero : Outport
  wires:
  Constant/1 -> Zero/1

== system CubeSatTEST/Real World/Hardware Models/Sensors/Sun Sensor (S4)/Mesurable (1) ==
  Action Port : ActionPort  ActionPortLabel=if((u1 == 0) & (u2 >= u3))
  Constant : Constant
  One : Outport
  wires:
  Constant/1 -> One/1

== system CubeSatTEST/Real World/Hardware Models/Sensors/Sun Sensor (S4)/Not Mesurable (0) ==
  Action Port : ActionPort  ActionPortLabel=else
  Constant : Constant  Value=0
  Zero : Outport
  wires:
  Constant/1 -> Zero/1

== system CubeSatTEST/OBC/Guidance/Sun Pointing Guidance/Attitude Error/[q (-)]/Xi(q) ==
  In1 : Inport
  Demux : Demux
  Gain{,1..5} (6 alike) : Gain  Gain=-1
  Matrix Concatenate : Concatenate  NumInputs=3  Mode=Multidimensional array  ConcatenateDimension=2
  Matrix Concatenate1 : Concatenate  NumInputs=4  Mode=Multidimensional array
  Matrix Concatenate2 : Concatenate  NumInputs=4  Mode=Multidimensional array
  Matrix Concatenate3 : Concatenate  NumInputs=4  Mode=Multidimensional array
  Out1 : Outport
  wires:
  In1/1 -> Demux/1
  Demux/2 -> [q2]
  Demux/3 -> [q3]
  Demux/4 -> [q4]
  Demux/1 -> [q1]
  Matrix Concatenate/1 -> Out1/1
  Matrix Concatenate1/1 -> Matrix Concatenate/1
  Matrix Concatenate2/1 -> Matrix Concatenate/2
  Matrix Concatenate3/1 -> Matrix Concatenate/3
  Gain1/1 -> Matrix Concatenate2/4
  [q1] -> Matrix Concatenate2/3
  Gain/1 -> Matrix Concatenate1/4
  [q3] -> Matrix Concatenate1/2
  [q2] -> Matrix Concatenate3/1
  Gain5/1 -> Matrix Concatenate3/4
  [q4] -> Matrix Concatenate1/1
  [q4] -> Matrix Concatenate2/2
  [q4] -> Matrix Concatenate3/3
  [q3] -> Gain2/1
  [q3] -> Gain5/1
  [q2] -> Gain3/1
  [q2] -> Gain1/1
  [q1] -> Gain/1
  [q1] -> Gain4/1
  Gain3/1 -> Matrix Concatenate1/3
  Gain2/1 -> Matrix Concatenate2/1
  Gain4/1 -> Matrix Concatenate3/2

== system CubeSatTEST/OBC/Navigation1/Q method/q_opt computing/Adj 3x3/C11 ==
  In1 : Inport
  22 : Selector  NumberOfDimensions=2  InputPortWidth=3  IndexOptions=Index vector (dialog),Index vector (dialog)  Indices=2,2  OutputSizes=1,1
  23 : Selector  NumberOfDimensions=2  InputPortWidth=3  IndexOptions=Index vector (dialog),Index vector (dialog)  Indices=2,3  OutputSizes=1,1
  32 : Selector  NumberOfDimensions=2  InputPortWidth=3  IndexOptions=Index vector (dialog),Index vector (dialog)  Indices=3,2  OutputSizes=1,1
  33 : Selector  NumberOfDimensions=2  InputPortWidth=3  IndexOptions=Index vector (dialog),Index vector (dialog)  Indices=3,3  OutputSizes=1,1
  Product : Product
  Product1 : Product
  Subtract : Sum  Inputs=+-
  Out1 : Outport
  wires:
  In1/1 -> 32/1, 23/1, 33/1, 22/1
  22/1 -> Product/1
  33/1 -> Product/2
  23/1 -> Product1/1
  32/1 -> Product1/2
  Subtract/1 -> Out1/1
  Product/1 -> Subtract/1
  Product1/1 -> Subtract/2

== system CubeSatTEST/OBC/Navigation1/Q method/q_opt computing/Adj 3x3/C12 ==
  In1 : Inport
  21 : Selector  NumberOfDimensions=2  InputPortWidth=3  IndexOptions=Index vector (dialog),Index vector (dialog)  Indices=2,1  OutputSizes=1,1
  23 : Selector  NumberOfDimensions=2  InputPortWidth=3  IndexOptions=Index vector (dialog),Index vector (dialog)  Indices=2,3  OutputSizes=1,1
  31 : Selector  NumberOfDimensions=2  InputPortWidth=3  IndexOptions=Index vector (dialog),Index vector (dialog)  Indices=3,1  OutputSizes=1,1
  33 : Selector  NumberOfDimensions=2  InputPortWidth=3  IndexOptions=Index vector (dialog),Index vector (dialog)  Indices=3,3  OutputSizes=1,1
  Gain : Gain  Gain=-1
  Product : Product
  Product1 : Product
  Subtract : Sum  Inputs=+-
  Out1 : Outport
  wires:
  In1/1 -> 23/1, 31/1, 33/1, 21/1
  21/1 -> Product/1
  33/1 -> Product/2
  31/1 -> Product1/1
  23/1 -> Product1/2
  Subtract/1 -> Gain/1
  Product/1 -> Subtract/1
  Product1/1 -> Subtract/2
  Gain/1 -> Out1/1

== system CubeSatTEST/OBC/Navigation1/Q method/q_opt computing/Adj 3x3/C13 ==
  In1 : Inport
  21 : Selector  NumberOfDimensions=2  InputPortWidth=3  IndexOptions=Index vector (dialog),Index vector (dialog)  Indices=2,1  OutputSizes=1,1
  22 : Selector  NumberOfDimensions=2  InputPortWidth=3  IndexOptions=Index vector (dialog),Index vector (dialog)  Indices=2,2  OutputSizes=1,1
  31 : Selector  NumberOfDimensions=2  InputPortWidth=3  IndexOptions=Index vector (dialog),Index vector (dialog)  Indices=3,1  OutputSizes=1,1
  32 : Selector  NumberOfDimensions=2  InputPortWidth=3  IndexOptions=Index vector (dialog),Index vector (dialog)  Indices=3,2  OutputSizes=1,1
  Product : Product
  Product1 : Product
  Subtract : Sum  Inputs=+-
  Out1 : Outport
  wires:
  In1/1 -> 31/1, 22/1, 32/1, 21/1
  21/1 -> Product/1
  32/1 -> Product/2
  22/1 -> Product1/1
  31/1 -> Product1/2
  Subtract/1 -> Out1/1
  Product/1 -> Subtract/1
  Product1/1 -> Subtract/2

== system CubeSatTEST/OBC/Navigation1/Q method/q_opt computing/Adj 3x3/C21 ==
  In1 : Inport
  12 : Selector  NumberOfDimensions=2  InputPortWidth=3  IndexOptions=Index vector (dialog),Index vector (dialog)  Indices=1,2  OutputSizes=1,1
  13 : Selector  NumberOfDimensions=2  InputPortWidth=3  IndexOptions=Index vector (dialog),Index vector (dialog)  Indices=1,3  OutputSizes=1,1
  32 : Selector  NumberOfDimensions=2  InputPortWidth=3  IndexOptions=Index vector (dialog),Index vector (dialog)  Indices=3,2  OutputSizes=1,1
  33 : Selector  NumberOfDimensions=2  InputPortWidth=3  IndexOptions=Index vector (dialog),Index vector (dialog)  Indices=3,3  OutputSizes=1,1
  Gain : Gain  Gain=-1
  Product : Product
  Product1 : Product
  Subtract : Sum  Inputs=+-
  Out1 : Outport
  wires:
  In1/1 -> 32/1, 13/1, 33/1, 12/1
  12/1 -> Product/1
  33/1 -> Product/2
  13/1 -> Product1/1
  32/1 -> Product1/2
  Subtract/1 -> Gain/1
  Product/1 -> Subtract/1
  Product1/1 -> Subtract/2
  Gain/1 -> Out1/1

== system CubeSatTEST/OBC/Navigation1/Q method/q_opt computing/Adj 3x3/C22 ==
  In1 : Inport
  11 : Selector  NumberOfDimensions=2  InputPortWidth=3  IndexOptions=Index vector (dialog),Index vector (dialog)  Indices=1,1  OutputSizes=1,1
  13 : Selector  NumberOfDimensions=2  InputPortWidth=3  IndexOptions=Index vector (dialog),Index vector (dialog)  Indices=1,3  OutputSizes=1,1
  31 : Selector  NumberOfDimensions=2  InputPortWidth=3  IndexOptions=Index vector (dialog),Index vector (dialog)  Indices=3,1  OutputSizes=1,1
  33 : Selector  NumberOfDimensions=2  InputPortWidth=3  IndexOptions=Index vector (dialog),Index vector (dialog)  Indices=3,3  OutputSizes=1,1
  Product : Product
  Product1 : Product
  Subtract : Sum  Inputs=+-
  Out1 : Outport
  wires:
  In1/1 -> 31/1, 13/1, 33/1, 11/1
  11/1 -> Product/1
  33/1 -> Product/2
  13/1 -> Product1/1
  31/1 -> Product1/2
  Subtract/1 -> Out1/1
  Product/1 -> Subtract/1
  Product1/1 -> Subtract/2

== system CubeSatTEST/OBC/Navigation1/Q method/q_opt computing/Adj 3x3/C23 ==
  In1 : Inport
  11 : Selector  NumberOfDimensions=2  InputPortWidth=3  IndexOptions=Index vector (dialog),Index vector (dialog)  Indices=1,1  OutputSizes=1,1
  12 : Selector  NumberOfDimensions=2  InputPortWidth=3  IndexOptions=Index vector (dialog),Index vector (dialog)  Indices=1,2  OutputSizes=1,1
  31 : Selector  NumberOfDimensions=2  InputPortWidth=3  IndexOptions=Index vector (dialog),Index vector (dialog)  Indices=3,1  OutputSizes=1,1
  32 : Selector  NumberOfDimensions=2  InputPortWidth=3  IndexOptions=Index vector (dialog),Index vector (dialog)  Indices=3,2  OutputSizes=1,1
  Gain : Gain  Gain=-1
  Product : Product
  Product1 : Product
  Subtract : Sum  Inputs=+-
  Out1 : Outport
  wires:
  In1/1 -> 12/1, 31/1, 32/1, 11/1
  11/1 -> Product/1
  32/1 -> Product/2
  31/1 -> Product1/1
  12/1 -> Product1/2
  Subtract/1 -> Gain/1
  Product/1 -> Subtract/1
  Product1/1 -> Subtract/2
  Gain/1 -> Out1/1

== system CubeSatTEST/OBC/Navigation1/Q method/q_opt computing/Adj 3x3/C31 ==
  In1 : Inport
  12 : Selector  NumberOfDimensions=2  InputPortWidth=3  IndexOptions=Index vector (dialog),Index vector (dialog)  Indices=1,2  OutputSizes=1,1
  13 : Selector  NumberOfDimensions=2  InputPortWidth=3  IndexOptions=Index vector (dialog),Index vector (dialog)  Indices=1,3  OutputSizes=1,1
  22 : Selector  NumberOfDimensions=2  InputPortWidth=3  IndexOptions=Index vector (dialog),Index vector (dialog)  Indices=2,2  OutputSizes=1,1
  23 : Selector  NumberOfDimensions=2  InputPortWidth=3  IndexOptions=Index vector (dialog),Index vector (dialog)  Indices=2,3  OutputSizes=1,1
  Product : Product
  Product1 : Product
  Subtract : Sum  Inputs=+-
  Out1 : Outport
  wires:
  In1/1 -> 22/1, 13/1, 23/1, 12/1
  12/1 -> Product/1
  23/1 -> Product/2
  13/1 -> Product1/1
  22/1 -> Product1/2
  Subtract/1 -> Out1/1
  Product/1 -> Subtract/1
  Product1/1 -> Subtract/2

== system CubeSatTEST/OBC/Navigation1/Q method/q_opt computing/Adj 3x3/C32 ==
  In1 : Inport
  11 : Selector  NumberOfDimensions=2  InputPortWidth=3  IndexOptions=Index vector (dialog),Index vector (dialog)  Indices=1,1  OutputSizes=1,1
  13 : Selector  NumberOfDimensions=2  InputPortWidth=3  IndexOptions=Index vector (dialog),Index vector (dialog)  Indices=1,3  OutputSizes=1,1
  21 : Selector  NumberOfDimensions=2  InputPortWidth=3  IndexOptions=Index vector (dialog),Index vector (dialog)  Indices=2,1  OutputSizes=1,1
  23 : Selector  NumberOfDimensions=2  InputPortWidth=3  IndexOptions=Index vector (dialog),Index vector (dialog)  Indices=2,3  OutputSizes=1,1
  Gain : Gain  Gain=-1
  Product : Product
  Product1 : Product
  Subtract : Sum  Inputs=+-
  Out1 : Outport
  wires:
  In1/1 -> 21/1, 13/1, 23/1, 11/1
  11/1 -> Product/1
  23/1 -> Product/2
  13/1 -> Product1/1
  21/1 -> Product1/2
  Subtract/1 -> Gain/1
  Product/1 -> Subtract/1
  Product1/1 -> Subtract/2
  Gain/1 -> Out1/1

== system CubeSatTEST/OBC/Navigation1/Q method/q_opt computing/Adj 3x3/C33 ==
  In1 : Inport
  11 : Selector  NumberOfDimensions=2  InputPortWidth=3  IndexOptions=Index vector (dialog),Index vector (dialog)  Indices=1,1  OutputSizes=1,1
  12 : Selector  NumberOfDimensions=2  InputPortWidth=3  IndexOptions=Index vector (dialog),Index vector (dialog)  Indices=1,2  OutputSizes=1,1
  21 : Selector  NumberOfDimensions=2  InputPortWidth=3  IndexOptions=Index vector (dialog),Index vector (dialog)  Indices=2,1  OutputSizes=1,1
  22 : Selector  NumberOfDimensions=2  InputPortWidth=3  IndexOptions=Index vector (dialog),Index vector (dialog)  Indices=2,2  OutputSizes=1,1
  Product : Product
  Product1 : Product
  Subtract : Sum  Inputs=+-
  Out1 : Outport
  wires:
  In1/1 -> 21/1, 12/1, 22/1, 11/1
  11/1 -> Product/1
  22/1 -> Product/2
  12/1 -> Product1/1
  21/1 -> Product1/2
  Subtract/1 -> Out1/1
  Product/1 -> Subtract/1
  Product1/1 -> Subtract/2

== system CubeSatTEST/OBC/Navigation1/Q method/q_opt computing/Det 3x3/Adj 3x3 ==
  In1 : Inport
  C11 : Subsystem
  C12 : Subsystem
  C13 : Subsystem
  C21 : Subsystem
  C22 : Subsystem
  C23 : Subsystem
  C31 : Subsystem
  C32 : Subsystem
  C33 : Subsystem
  From{,1..8} (9 alike) : From
  Goto : Goto
  Matrix Concatenate : Concatenate  NumInputs=3  Mode=Multidimensional array
  Matrix Concatenate1 : Concatenate  NumInputs=3  Mode=Multidimensional array
  Matrix Concatenate2 : Concatenate  NumInputs=3  Mode=Multidimensional array
  Matrix Concatenate3 : Concatenate  NumInputs=3  Mode=Multidimensional array  ConcatenateDimension=2
  Transpose : Math  Operator=transpose
  Out1 : Outport
  wires:
  Transpose/1 -> Out1/1
  In1/1 -> Goto/1
  C11/1(Out1) -> Matrix Concatenate/1
  C21/1(Out1) -> Matrix Concatenate/2
  C31/1(Out1) -> Matrix Concatenate/3
  C22/1(Out1) -> Matrix Concatenate1/2
  C12/1(Out1) -> Matrix Concatenate1/1
  C32/1(Out1) -> Matrix Concatenate1/3
  C23/1(Out1) -> Matrix Concatenate2/2
  C13/1(Out1) -> Matrix Concatenate2/1
  C33/1(Out1) -> Matrix Concatenate2/3
  Matrix Concatenate3/1 -> Transpose/1
  Matrix Concatenate2/1 -> Matrix Concatenate3/3
  Matrix Concatenate1/1 -> Matrix Concatenate3/2
  Matrix Concatenate/1 -> Matrix Concatenate3/1
  From/1 -> C11/1(In1)
  From1/1 -> C21/1(In1)
  From2/1 -> C31/1(In1)
  From3/1 -> C22/1(In1)
  From4/1 -> C32/1(In1)
  From5/1 -> C12/1(In1)
  From6/1 -> C13/1(In1)
  From7/1 -> C23/1(In1)
  From8/1 -> C33/1(In1)

== system CubeSatTEST/OBC/Navigation1/Q method/q_opt computing/||q||1/[q (x)] ==
  In1 : Inport
  Matrix Concatenate : Concatenate  Mode=Multidimensional array  ConcatenateDimension=2
  Psi(q) : Subsystem
  Out1 : Outport
  wires:
  Psi(q)/1(Out1) -> Matrix Concatenate/1
  In1/1 -> Matrix Concatenate/2, Psi(q)/1(In1)
  Matrix Concatenate/1 -> Out1/1

== system CubeSatTEST/OBC/Navigation1/Q method/q_opt computing/||q||1/q* ==
  note: Evaluate the quaternion coniugate
  q : Inport
  Demux : Demux
  Gain : Gain  Gain=-1
  Gain1 : Gain  Gain=-1
  Gain2 : Gain  Gain=-1
  Mux : Mux
  q* : Outport
  wires:
  Gain2/1 -> Mux/3
  Gain1/1 -> Mux/2
  Gain/1 -> Mux/1
  Demux/3 -> Gain2/1
  Demux/2 -> Gain1/1
  Demux/1 -> Gain/1
  q/1 -> Demux/1
  Demux/4 -> Mux/4
  Mux/1 -> q*/1

== system CubeSatTEST/OBC/Navigation1/Sequential Rotations/Q method/S and Z matrix computing/Trace ==
  In1 : Inport
  Extract Diagonal : matrix_library/Extract Diagonal
  Sum of Elements : Sum  Inputs=+
  Out1 : Outport
  wires:
  In1/1 -> Extract Diagonal/1
  Extract Diagonal/1 -> Sum of Elements/1
  Sum of Elements/1 -> Out1/1

== system CubeSatTEST/OBC/Navigation1/Sequential Rotations/Q method/Subsystem/Norm1 ==
  Vector : Inport
  Add : Sum  Inputs=+++
  Demux : Demux  Outputs=3
  Sqrt : Sqrt
  Square : Math  Operator=square
  Square1 : Math  Operator=square
  Square2 : Math  Operator=square
  Norm : Outport
  wires:
  Square/1 -> Add/1
  Add/1 -> Sqrt/1
  Demux/3 -> Square1/1
  Square2/1 -> Add/2
  Square1/1 -> Add/3
  Demux/1 -> Square/1
  Demux/2 -> Square2/1
  Vector/1 -> Demux/1
  Sqrt/1 -> Norm/1

== system CubeSatTEST/OBC/Navigation1/Sequential Rotations/Q method/Subsystem/Norm2 ==
  Vector : Inport
  Add : Sum  Inputs=+++
  Demux : Demux  Outputs=3
  Sqrt : Sqrt
  Square : Math  Operator=square
  Square1 : Math  Operator=square
  Square2 : Math  Operator=square
  Norm : Outport
  wires:
  Square/1 -> Add/1
  Add/1 -> Sqrt/1
  Demux/3 -> Square1/1
  Square2/1 -> Add/2
  Square1/1 -> Add/3
  Demux/1 -> Square/1
  Demux/2 -> Square2/1
  Vector/1 -> Demux/1
  Sqrt/1 -> Norm/1

== system CubeSatTEST/OBC/Navigation1/Sequential Rotations/Q method/q_opt computing/Adj 3x3 ==
  A : Inport
  C11 : Subsystem
  C12 : Subsystem
  C13 : Subsystem
  C21 : Subsystem
  C22 : Subsystem
  C23 : Subsystem
  C31 : Subsystem
  C32 : Subsystem
  C33 : Subsystem
  From{,1..8} (9 alike) : From
  Goto : Goto
  Matrix Concatenate : Concatenate  NumInputs=3  Mode=Multidimensional array
  Matrix Concatenate1 : Concatenate  NumInputs=3  Mode=Multidimensional array
  Matrix Concatenate2 : Concatenate  NumInputs=3  Mode=Multidimensional array
  Matrix Concatenate3 : Concatenate  NumInputs=3  Mode=Multidimensional array  ConcatenateDimension=2
  Transpose : Math  Operator=transpose
  Adj(A) : Outport
  wires:
  Transpose/1 -> Adj(A)/1
  A/1 -> Goto/1
  C11/1(Out1) -> Matrix Concatenate/1
  C21/1(Out1) -> Matrix Concatenate/2
  C31/1(Out1) -> Matrix Concatenate/3
  C22/1(Out1) -> Matrix Concatenate1/2
  C12/1(Out1) -> Matrix Concatenate1/1
  C32/1(Out1) -> Matrix Concatenate1/3
  C23/1(Out1) -> Matrix Concatenate2/2
  C13/1(Out1) -> Matrix Concatenate2/1
  C33/1(Out1) -> Matrix Concatenate2/3
  Matrix Concatenate3/1 -> Transpose/1
  Matrix Concatenate2/1 -> Matrix Concatenate3/3
  Matrix Concatenate1/1 -> Matrix Concatenate3/2
  Matrix Concatenate/1 -> Matrix Concatenate3/1
  From/1 -> C11/1(In1)
  From1/1 -> C21/1(In1)
  From2/1 -> C31/1(In1)
  From3/1 -> C22/1(In1)
  From4/1 -> C32/1(In1)
  From5/1 -> C12/1(In1)
  From6/1 -> C13/1(In1)
  From7/1 -> C23/1(In1)
  From8/1 -> C33/1(In1)

== system CubeSatTEST/OBC/Navigation1/Sequential Rotations/Q method/q_opt computing/Det 3x3 ==
  A : Inport
  Adj 3x3 : Subsystem
  Matrix Multiply : Product  Multiplication=Matrix(*)
  Selector : Selector  NumberOfDimensions=2  InputPortWidth=3  IndexOptions=Index vector (dialog),Index vector (dialog)  Indices=1,1  OutputSizes=1,1
  det(A) : Outport
  wires:
  A/1 -> Adj 3x3/1(In1), Matrix Multiply/1
  Adj 3x3/1(Out1) -> Matrix Multiply/2
  Matrix Multiply/1 -> Selector/1
  Selector/1 -> det(A)/1

== system CubeSatTEST/OBC/Navigation1/Sequential Rotations/Q method/q_opt computing/Trace ==
  B : Inport
  Extract Diagonal : matrix_library/Extract Diagonal
  Sum of Elements : Sum  Inputs=+
  tr(B) : Outport
  wires:
  B/1 -> Extract Diagonal/1
  Extract Diagonal/1 -> Sum of Elements/1
  Sum of Elements/1 -> tr(B)/1
